simulink model "motor_ideal"  (R2013a)
settings: Solver=ode45  StartTime=0.0  StopTime=inf  RelTol=1e-3
values from neighbouring files (symbols this model uses):
  b = 0.1    [data_ideal_motor_1.mat]    (also in identificacion2.m)
  id_motor =     [LAB02_IDENT.mat]    (also in LAB02_IDENT_02.mat; data_ideal_motor_1.mat)
  J = 0.01    [data_ideal_motor_1.mat]    (also in identificacion2.m)
  K = K1    (= 1.59952738349)    [bodes.m]    (also in data_ideal_motor_1.mat = 0.01; identificacion2.m = 0.01)
  L = 0.5    [data_ideal_motor_1.mat]    (also in identificacion2.m)
  R = 1    [data_ideal_motor_1.mat]    (also in identificacion2.m)
libraries: dsparch4 x1
settings Model: Creator=u_labelectro  LastModifiedBy=u_labelectro
settings HardwareCC: ProdIntDivRoundTo=Zero  ProdEndianess=LittleEndian  ProdHWDeviceType=Generic->32-bit x86 compatible
settings RTWCC: SystemTargetFile=rtwin.tlc  TemplateMakefile=rtwin.tmf  Description=Real-Time Windows Target  ProcessScript=rtwin_make_rtw_hook  RTWCompilerOptimization=On
settings CodeAppCC: MaxIdLength=95
settings RTWinTargetCC: TargetLibSuffix=_rtwin.lib  TargetPreCompLibLocation=D:\Real Time\toolbox\rtw\targets\rtwin\lib\win64  CodeReplacementLibrary=ANSI_C  RTWinDir=D:/REALTI~1/toolbox/rtw/targets/rtwin  TargetArch=win64

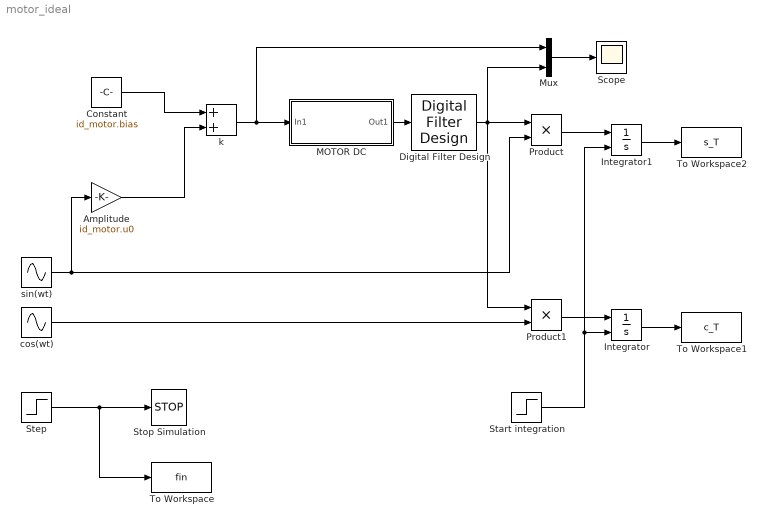
== system motor_ideal ==
  Amplitude : Gain  Gain=id_motor.u0
  Constant : Constant  Value=id_motor.bias
  Digital Filter Design : dsparch4/Digital Filter Design  mwdsp_browser_bugfix_var=off
  Integrator : Integrator  ExternalReset=rising
  Integrator1 : Integrator  ExternalReset=rising
  "MOTOR DC " : Subsystem  TreatAsAtomicUnit=on
  Mux : Mux  Inputs=2
  Product : Product
  Product1 : Product
  Scope : Scope
      settings: TimeRange=10  YMin=-10  YMax=10
  Start integration : Step  Time=id_motor.Tstart  SampleTime=0
  Step : Step  Time=id_motor.Tstop  SampleTime=0
  Stop Simulation : Stop
  To Workspace : ToWorkspace  VariableName=fin  SampleTime=-1  SaveFormat=Timeseries
  To Workspace1 : ToWorkspace  VariableName=c_T  SampleTime=-1
  To Workspace2 : ToWorkspace  VariableName=s_T  SampleTime=-1
  cos(wt) : Sin  Frequency=id_motor.w  Phase=pi/2  Samples=id_motor.w/id_motor.s  SampleTime=id_motor.s  Offset=5
  k : Sum
  sin(wt) : Sin  Frequency=id_motor.w  Samples=(id_motor.w)/(id_motor.s)  SampleTime=id_motor.s
  wires:
  Step/1 -> To Workspace/1, Stop Simulation/1
  Constant/1 -> k/1
  Amplitude/1 -> k/2
  Digital Filter Design/1 -> Mux/2, Product/1, Product1/1
  k/1 -> "MOTOR DC "/1(In1), Mux/1
  Product/1 -> Integrator1/1
  Product1/1 -> Integrator/1
  Start integration/1 -> Integrator/2, Integrator1/2
  sin(wt)/1 -> Amplitude/1, Product/2
  cos(wt)/1 -> Product1/2
  Integrator1/1 -> To Workspace2/1
  Integrator/1 -> To Workspace1/1
  Mux/1 -> Scope/1
  "MOTOR DC "/1(Out1) -> Digital Filter Design/1

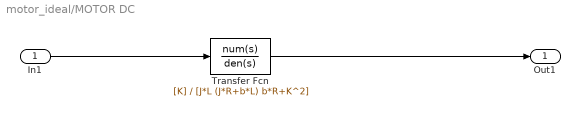
== system motor_ideal/MOTOR DC  ==
  In1 : Inport
  Transfer Fcn : TransferFcn  Numerator=[K]  Denominator=[J*L (J*R+b*L) b*R+K^2]
  Out1 : Outport
  wires:
  Transfer Fcn/1 -> Out1/1
  In1/1 -> Transfer Fcn/1
